simulink model "simulink_q2"  (R2022b)
settings: Solver=VariableStepAuto  StartTime=0.0  StopTime=10.0  RelTol=1e-3
settings Model: Creator=NITRO  LastModifiedBy=NITRO

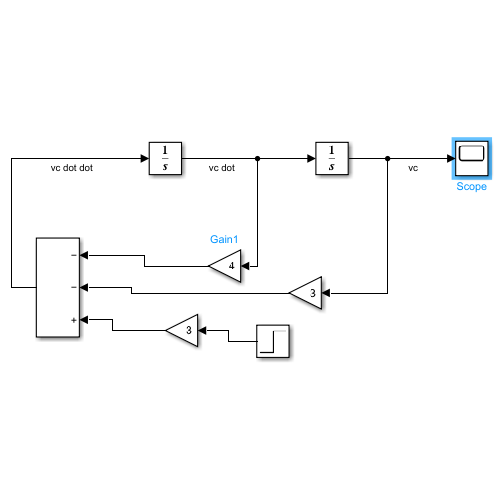
[thumbnail: Simulink's stored preview of the top-level diagram]
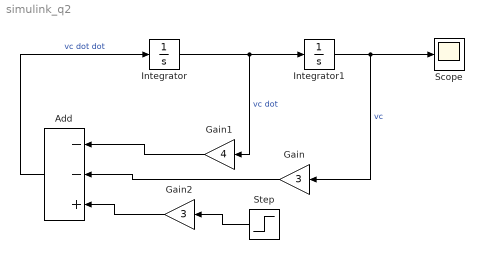
== system simulink_q2 ==
  Add : Sum  Inputs=--+
  Gain : Gain  Gain=3
  Gain1 : Gain  Gain=4
  Gain2 : Gain  Gain=3
  Integrator : Integrator
  Integrator1 : Integrator  InitialCondition=0.5
  Scope : Scope
  Step : Step  SampleTime=0
  wires:
  Integrator/1 -> Gain1/1, Integrator1/1  "vc dot"
  Add/1 -> Integrator/1  "vc dot dot"
  Integrator1/1 -> Gain/1, Scope/1  "vc"
  Gain1/1 -> Add/1
  Gain/1 -> Add/2
  Step/1 -> Gain2/1
  Gain2/1 -> Add/3
